simulink model "System_noSolution"  (R2023a)
settings: Solver=VariableStepAuto  StartTime=0.0  StopTime=100  RelTol=1e-3
undefined symbols (not defined in the file or in its folder): A, n_cal, R_mgt
libraries: dspsrcs4 x1
settings Model: Creator=Personal  LastModifiedBy=Personal

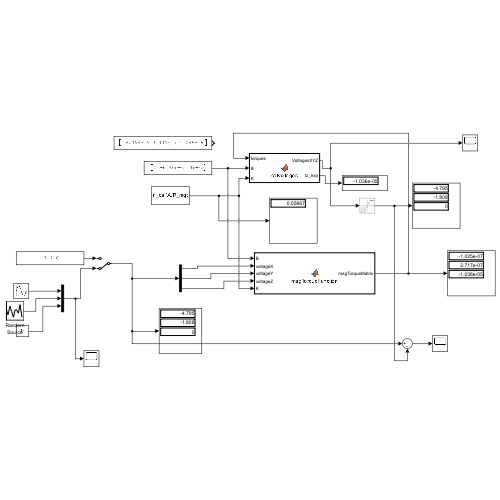
[thumbnail: Simulink's stored preview of the top-level diagram]
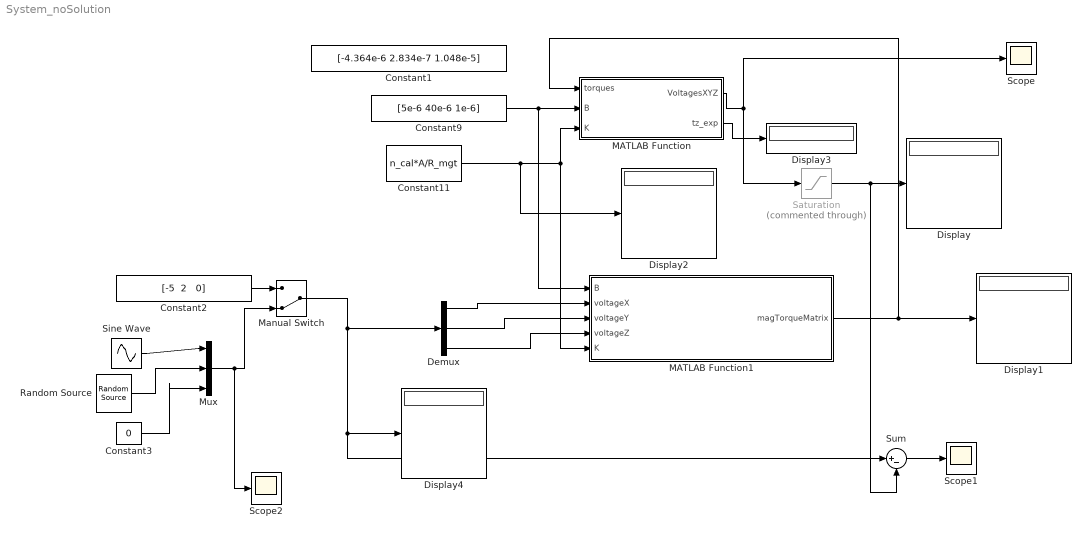
== system System_noSolution ==
  Constant1 : Constant  Value=[-4.364e-6 2.834e-7 1.048e-5]
  Constant11 : Constant  Value=n_cal*A/R_mgt
  Constant2 : Constant  Value="[-5  2   0]"
  Constant3 : Constant  Value=0
  Constant9 : Constant  Value=[5e-6 40e-6 1e-6]
  Demux : Demux  Outputs=3
  Display{,1..4} (5 alike) : Display
  MATLAB Function : MATLAB Function  TreatAsAtomicUnit=on
  MATLAB Function1 : MATLAB Function  TreatAsAtomicUnit=on
  Manual Switch : ManualSwitch  CurrentSetting=0
  Mux : Mux  Inputs=3
  Random Source : dspsrcs4/Random Source  SrcType=Uniform  NormMethod=Ziggurat  CltLength=12  MinVal=-5  MaxVal=5  MeanVal=0  VarVal=1  RepMode=Not repeatable  rawSeed=1  IsInherit=off  SampMode=Discrete  SampTime=1  SampFrame=1  DataType=Double  OutComplex=Real  OutputFrames=off
  Saturation : Saturate  Commented=through  UpperLimit=5  LowerLimit=-5
  Scope : Scope
  Scope1 : Scope
  Scope2 : Scope
  Sine Wave : Sin  Amplitude=5  Frequency=0.05  SampleTime=0
  Sum : Sum  Inputs=|+-
  wires:
  Constant11/1 -> Display2/1, MATLAB Function1/5(K), MATLAB Function/3(K)
  Constant9/1 -> MATLAB Function1/1(B), MATLAB Function/2(B)
  MATLAB Function/1(VoltagesXYZ) -> Saturation/1, Scope/1
  Saturation/1 -> Sum/2, Display/1
  Demux/1 -> MATLAB Function1/2(voltageX)
  Demux/2 -> MATLAB Function1/3(voltageY)
  Demux/3 -> MATLAB Function1/4(voltageZ)
  Manual Switch/1 -> Display4/1, Sum/1, Demux/1
  MATLAB Function1/1(magTorqueMatrix) -> MATLAB Function/1(torques), Display1/1
  MATLAB Function/2(tz_exp) -> Display3/1
  Sum/1 -> Scope1/1
  Constant2/1 -> Manual Switch/1
  Mux/1 -> Scope2/1, Manual Switch/2
  Constant3/1 -> Mux/3
  Sine Wave/1 -> Mux/1
  Random Source/1 -> Mux/2

== matlab function System_noSolution/MATLAB Function1 ==
  data: B input; magTorqueMatrix output; voltageX input; voltageY input; voltageZ input; K input
function magTorqueMatrix  = magTorqueFunction(B,voltageX,voltageY,voltageZ,K)




magTorqueMatrix_X = cross(voltageX*K*[1 0 0],B);
magTorqueMatrix_Y = cross(voltageY*K*[0 1 0],B);
magTorqueMatrix_Z = cross(voltageZ*K*[0 0 1],B);
 

magTorqueMatrix = magTorqueMatrix_X+magTorqueMatrix_Y+magTorqueMatrix_Z;

== matlab function System_noSolution/MATLAB Function ==
  data: torques input; VoltagesXYZ output; B input; K input; tz_exp output
function [VoltagesXYZ,tz_exp] = calVoltages(torques,B,K)
Bx = B(1);
By = B(2);
Bz = B(3);

Tx = torques(1);
Ty = torques(2);
Tz = torques(3);


% % syms Vx Vy Vz
% % eqn1 = 0*Vx + K*Bz*Vy -K*By*Vz == Tx;
% % eqn2 = -K*Bz*Vx + 0*Vy +K*Bx*Vz == Ty;
% % eqn3 = K*By*Vx -K*Bx*Vy +0*Vz == Tz;
% % 
% % [A,B] = equationsToMatrix([eqn1, eqn2, eqn3], [Vx, Vy, Vz]);
% 
% A = [0 K*Bz -K*By;
%     -K*Bz 0 K*Bx;
%     K*By -K*Bx 0];
% B = torques;
% 
% VoltagesXYZ = A^-1*B;
Vx = -Ty/(K*Bz);
Vy = Tx/(K*Bz);
tz_exp = -(By/Bz)*Ty-(Bx/Bz)*Tx;

VoltagesXYZ = [Vx Vy 0];
end
